simulink model "CellCharacterizationHPPC"  (R2023b)
settings: Solver=ode1be  StartTime=0.0  StopTime=100000  FixedStep=1  MaxStep=1  RelTol=1e-3  AbsTol=1e-3
PreLoadFcn:
  | createHPPCprofile = load('origCellDataHPPCdataGen.mat');
libraries: fl_lib x2, nesl_utility x2, batteryecm_lib x1
settings Model: Creator=The MathWorks, Inc.  LastModifiedBy=jjha
settings SolverCC: AutoScaleAbsTol=off  AlgebraicLoopSolver=TrustRegion  MaxZcPerStep=1
settings DataIOCC: ReturnWorkspaceOutputsName=batt_BatteryCellCharacterizationForBEV_HPPC
settings OptimizationCC: ReuseModelBlockBuffer=off
settings DebuggingCC: UnconnectedInputMsg=warning  UnconnectedOutputMsg=warning  UnconnectedLineMsg=warning  SymbolicDimsDataTypeCodeGenerationDiagnostic=none
settings ModelReferenceCC: EnableRefExpFcnMdlSchedulingChecks=on
settings SFSimCC: CustomCodeUndefinedFunction=UseInterfaceOnly
settings RTWCC: DLArmComputeVersion=19.05
settings SimscapeCC: SimscapeLogType=all  SimscapeLogSimulationStatistics=on  SimscapeLogName=simlog_CellCharacterizationHPPC  SimscapeLogDataHistory=10000

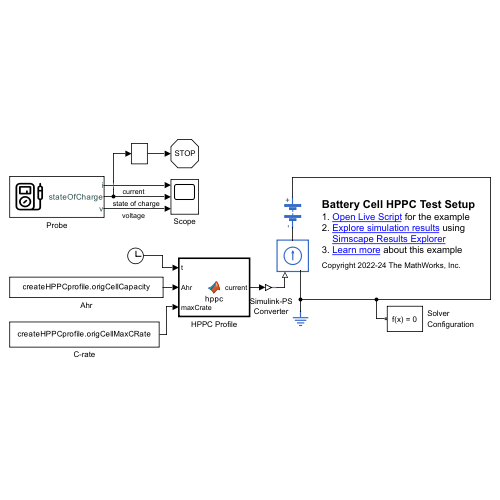
[thumbnail: Simulink's stored preview of the top-level diagram]
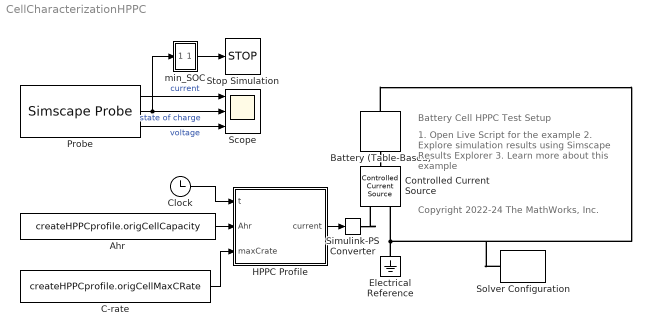
== system CellCharacterizationHPPC ==
  note: Battery Cell HPPC Test Setup
  note: 1. Open Live Script for the example
      | 2. Explore simulation results using
      | Simscape Results Explorer
      | 3. Learn more about this example
  note: Copyright 2022-24 The MathWorks, Inc.
  Ahr : Constant  Value=createHPPCprofile.origCellCapacity
  Battery (Table-Based) : batteryecm_lib/Battery (Table-Based)  SOC_vec=createHPPCprofile.origCellData.SOC  T_dependence=simscape.enum.tablebattery.temperature_dependence.no  prm_dir=simscape.enum.tablebattery.prm_dir.currentDirectionality  T_vec=[278, 293, 313] K  V0_mat=[3.49, 3.5, 3.51; 3.55, 3.57, 3.56; 3.62, 3.63, 3.64; 3.71, 3.71, 3.72; 3.91, 3.93, 3.94; 4.07, 4.08, 4.08; 4.19, 4.19, 4.19] V  V0_vec=createHPPCprofile.origCellData.V0 V  V_range=[0, inf] V  R0_mat=[.0117, .0085, .009; .011, .0085, .009; .0114, .0087, .0092; .0107, .0082, .0088; .0107, .0083, .0091; .0113, .0085, .0089; .0116, .0085, .0089] Ohm  R0_vec=origCell.R0 Ohm  R0_dis_mat=[.0117, .0085, .009; .011, .0085, .009; .0114, .0087, .0092; .0107, .0082, .0088; .0107, .0083, .0091; .0113, .0085, .0089; .0116, .0085, .0089] Ohm  R0_dis_vec=createHPPCprofile.origCellData.R0discharge Ohm  R0_ch_mat=[.0117, .0085, .009; .011, .0085, .009; .0114, .0087, .0092; .0107, .0082, .0088; .0107, .0083, .0091; .0113, .0085, .0089; .0116, .0085, .0089] Ohm  R0_ch_vec=createHPPCprofile.origCellData.R0charge Ohm  AH=createHPPCprofile.origCellCapacity A*hr  prm_leak=simscape.enum.tablebattery.prm_leak.disabled  Rleak_vec=[8000, 7000, 6000] Ohm  Rleak=7e3 Ohm  extrapolation_option=simscape.enum.extrapolation.nearest  SOC_port=simscape.enum.tablebattery.enable.no  prm_dyn=simscape.enum.tablebattery.prm_dyn.rc3  R1_mat=[.0109, .0029, .0013; .0069, .0024, .0012; .0047, .0026, .0013; .0034, .0016, .001; .0033, .0023, .0014; .0033, .0018, .0011; .0028, .0017, .0011] Ohm  R1_vec=createHPPCprofile.origCellData.R1rest Ohm  tau1_mat=[20, 36, 39; 31, 45, 39; 109, 105, 61; 36, 29, 26; 59, 77, 67; 40, 33, 29; 25, 39, 33] s  tau1_vec=createHPPCprofile.origCellData.Tau1rest s  R2_mat=[.0109, .0029, .0013; .0069, .0024, .0012; .0047, .0026, .0013; .0034, .0016, .001; .0033, .0023, .0014; .0033, .0018, .0011; .0028, .0017, .0011] Ohm  R2_vec=createHPPCprofile.origCellData.R2rest Ohm  tau2_mat=[20, 36, 39; 31, 45, 39; 109, 105, 61; 36, 29, 26; 59, 77, 67; 40, 33, 29; 25, 39, 33] s  tau2_vec=createHPPCprofile.origCellData.Tau2rest s  R3_mat=[.0109, .0029, .0013; .0069, .0024, .0012; .0047, .0026, .0013; .0034, .0016, .001; .0033, .0023, .0014; .0033, .0018, .0011; .0028, .0017, .0011] Ohm  R3_vec=createHPPCprofile.origCellData.R3rest Ohm  tau3_mat=[20, 36, 39; 31, 45, 39; 109, 105, 61; 36, 29, 26; 59, 77, 67; 40, 33, 29; 25, 39, 33] s  tau3_vec=createHPPCprofile.origCellData.Tau3rest s  R4_mat=[.0109, .0029, .0013; .0069, .0024, .0012; .0047, .0026, .0013; .0034, .0016, .001; .0033, .0023, .0014; .0033, .0018, .0011; .0028, .0017, .0011] Ohm  R4_vec=[.0029, .0024, .0026, .0016, .0023, .0018, .0017] Ohm  tau4_mat=[20, 36, 39; 31, 45, 39; 109, 105, 61; 36, 29, 26; 59, 77, 67; 40, 33, 29; 25, 39, 33] s  tau4_vec=[36, 45, 105, 29, 77, 33, 39] s  R5_mat=[.0109, .0029, .0013; .0069, .0024, .0012; .0047, .0026, .0013; .0034, .0016, .001; .0033, .0023, .0014; .0033, .0018, .0011; .0028, .0017, .0011] Ohm  R5_vec=[.0029, .0024, .0026, .0016, .0023, .0018, .0017] Ohm  tau5_mat=[20, 36, 39; 31, 45, 39; 109, 105, 61; 36, 29, 26; 59, 77, 67; 40, 33, 29; 25, 39, 33] s  tau5_vec=[36, 45, 105, 29, 77, 33, 39] s  prm_fade=simscape.enum.tablebattery.prm_fade.disabled  N0=100  dV0=0  dR0=0  dAH=0  dRleak=0  dR1=0  dR2=0  dR3=0  dR4=0  dR5=0  N0vec=[100, 200, 300]  Tfadevec=[298.15, 323.15] K  dV0vec=[0, 0, 0]  dR0vec=[0, 0, 0]  dAHvec=[0, 0, 0]  dRleakvec=[0, 0, 0]  dR1vec=[0, 0, 0]  dR2vec=[0, 0, 0]  dR3vec=[0, 0, 0]  dR4vec=[0, 0, 0]  dR5vec=[0, 0, 0]  dV0mat=[0, 0; 0, 0; 0, 0]  dR0mat=[0, 0; 0, 0; 0, 0]  dAHmat=[0, 0; 0, 0; 0, 0]  dRleakmat=[0, 0; 0, 0; 0, 0]  dR1mat=[0, 0; 0, 0; 0, 0]  dR2mat=[0, 0; 0, 0; 0, 0]  dR3mat=[0, 0; 0, 0; 0, 0]  dR4mat=[0, 0; 0, 0; 0, 0]  dR5mat=[0, 0; 0, 0; 0, 0]  prm_age_modeling=simscape.enum.tablebattery.prm_age_modeling.equation  storage_dt_age_vec=[0] d  storage_T_age_vec=[273] K  prm_age_OCV=simscape.enum.tablebattery.prm_age_OCV.OCV  OCV_age=0.9  SOC_age=0.6  prm_age_resistance=simscape.enum.tablebattery.prm_age.disabled  OCV_scaling_age_resistance=2.2134e6  OCV_offset_age_resistance=1.632e6  temp_exp_age_resistance=0.515833569 V  t_exp_age_resistance=0.75  T_age_vec_resistance=[273.15, 298.15, 323.15] K  dt_age_vec_resistance=[90, 180, 270, 360] d  dR0_age_vec=[0, 0, 0]  t_meas_dR0_age=100 d  dR0_age_mat=[0, 0, 0; 0, 0, 0; 0, 0, 0; 0, 0, 0]  prm_age_capacity=simscape.enum.tablebattery.prm_age.disabled  OCV_scaling_age_capacity=1.5097e07  OCV_offset_age_capacity=8.3625e06  temp_exp_age_capacity=0.6011 V  t_exp_age_capacity=0.75  T_age_vec_capacity=[273.15, 298.15, 323.15] K  dt_age_vec_capacity=[90, 180, 270, 360] d  dAH_age_vec=[0, 0, 0]  t_meas_dAH_age=100 d  dAH_age_mat=[0, 0, 0; 0, 0, 0; 0, 0, 0; 0, 0, 0]  thermal_port=simscape.enum.thermaleffects.omit  temperature=298.15 K  thermal_mass=100 J/K  i_specify=off  i_priority=None  i=0 A  i_nominal_specify=off  i_nominal_unit=A  i_nominal_value=1  v_specify=off  v_priority=None  v=0 V  v_nominal_specify=off  v_nominal_unit=V  v_nominal_value=1  stateOfCharge_specify=off  stateOfCharge_priority=High  stateOfCharge=1  stateOfCharge_nominal_specify=off  stateOfCharge_nominal_unit=1  stateOfCharge_nominal_value=1  num_cycles_specify=off  num_cycles_priority=High  num_cycles=0  num_cycles_nominal_specify=off  num_cycles_nominal_unit=1  num_cycles_nominal_value=1  cell_temperature_specify=off  cell_temperature_priority=High  cell_temperature=298.15 K  cell_temperature_nominal_specify=off  cell_temperature_nominal_unit=K  cell_temperature_nominal_value=1
      settings: InternalSimscapePortConfiguration="{\"Bottom\":[],\"Left\":[{\"id\":\"p\",\"label\":\"+\",\"type\":\"foundation.electrical.electrical\"}],\"Right\":[{\"id\":\"n\",\"label\":\"-\",\"type\":\"foundation.electrical.electrical\"}],\"Top\":[]}"
      settings: LibrarySourceBlock=|
      | batt_lib/Cells/Battery
      | (Table-Based)
  C-rate : Constant  Value=createHPPCprofile.origCellMaxCRate
  Clock : Clock
  Controlled Current Source : fl_lib/Electrical/Electrical Sources/Controlled Current Source
  Electrical Reference : fl_lib/Electrical/Electrical Elements/Electrical Reference
  HPPC Profile : MATLAB Function  TreatAsAtomicUnit=on
  Probe : SimscapeProbe  BoundBlock=22  Variables={i, stateOfCharge, v}
  Scope : Scope  NumInputPorts=3
  Simulink-PS Converter : nesl_utility/Simulink-PS Converter  PhysicalDomain=network_engine_domain  SubClassName=ps_input  LeftPortType=input  RightPortType=output  PseudoPeriodic=off  Frequencies=[]  NoiseDistribution=none  NoiseParameters=[]  Unit=A  AffineConversion=off  FilteringAndDerivatives=provide  SimscapeFilterOrder=1  InputFilterTimeConstant=0.001  UdotUserProvided=0
  Solver Configuration : nesl_utility/Solver Configuration  PhysicalDomain=network_engine_domain  SubClassName=solver  LeftPortType=input  RightPortType=generic  Tones=[]  Harmonics=[]  SimulateNoise=off  Profile=off  UseLocalSampling=off  EnableSwitchedLinearOptims=on  FrequencyDomain=off  UseCCode=off  RelTol=0.001  AbsTol=1e-06  MinStep=1e-09  ToWorkspace=off  RevertToSquareIcSolve=off  NumHomotopyIterations=100  PhasorMode=off  PhasorModeNumHarmonics=1  ConsistencySolver=NEWTON_XTOL_AFTER_FTOL  IndexReductionMethod=DerivativeReplacement  DoDC=off  ResidualTolerance=1e-09  ConsistencyTolSource=GLOBAL  ConsistencyAbsTol=0.001  ConsistencyRelTol=0.001  ConsistencyTolFactor=0.001  UseLocalSolver=off  LocalSolverChoice=NE_BACKWARD_EULER_ADVANCER  ResolveIndetEquations=on  FunctionEvalNumThread=1  LocalSolverSampleTime=0.001  DoFixedCost=off  MaxNonlinIter=3  MaxModeIter=2  ComputeImpulses=off  ImpulseIterations=2  LinearAlgebra=auto  LinearAlgebraNumThread=0  EquationFormulation=NE_TIME_EF  DelaysMemoryBudget=1024  AutomaticFiltering=on  FilteringTimeConstant=0.001  PartitionStorageMethod=AS_NEEDED  PartitionMemoryBudget=1024  PartitionMethod=ROBUST  MultibodyUseLocalSolver=off  MultibodyLocalSolverChoice=ODE1  MultibodyLocalSolverSampleTime=0.001
  Stop Simulation : Stop
  min_SOC : Subsystem
  wires:
  Probe/1 -> Scope/1  "current"
  Probe/2 -> min_SOC/1(" "), Scope/2  "state of charge"
  Probe/3 -> Scope/3  "voltage"
  Clock/1 -> HPPC Profile/1(t)
  HPPC Profile/1(current) -> Simulink-PS Converter/1
  Ahr/1 -> HPPC Profile/2(Ahr)
  min_SOC/1("  ") -> Stop Simulation/1
  C-rate/1 -> HPPC Profile/3(maxCrate)
  connections:
  Battery (Table-Based)/RConn1 -- Controlled Current Source/LConn1
  Simulink-PS Converter/RConn1 -- Controlled Current Source/RConn1
  Electrical Reference/LConn1 -- Controlled Current Source/RConn2 -- Solver Configuration/RConn1 -- Battery (Table-Based)/LConn1

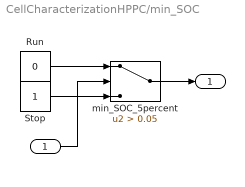
== system CellCharacterizationHPPC/min_SOC ==
  " " : Inport
  Run : Constant  Value=0
  Stop : Constant
  min_SOC_5percent : Switch  Criteria=u2 > Threshold  Threshold=0.05  SaturateOnIntegerOverflow=off  InputSameDT=off
  "  " : Outport
  wires:
  Run/1 -> min_SOC_5percent/1
  Stop/1 -> min_SOC_5percent/3
  " "/1 -> min_SOC_5percent/2
  min_SOC_5percent/1 -> "  "/1

== matlab function CellCharacterizationHPPC/HPPC Profile ==
  data: t input; current output; Ahr input; maxCrate input
function current = hppc(t,Ahr,maxCrate)
    dischg = -1; 
    chg = 1;
    cc_rate = 1/3;
    max_c_rate = maxCrate;
    %% Define HPPC protocol
    Imax = Ahr*max_c_rate; % Cell supplier provided maximum current that 
                           % can be passed through a cell, at a given 
                           % temperature
    const_curr_dischg= Ahr*cc_rate;% C/3 rate for moving to next SOC point
    pulse_chg_mag    = 0.75 * Imax;% Magnitude of charge pulse current
    pulse_dischg_mag = Imax;       % Magnitude of discharge pulse current
    pulse_time_gap   = 40;         % Rest time between charge and discharge 
                                   % pulses, in seconds
    pulse_chg_dur    = 10;         % Duration of charge pulse, in seconds
    pulse_dischg_dur = 30;         % Duration of discharge pulse, in seconds
    rest_time        = 3600;       % 2/3rd hour rest post charge-discharge 
                                   % pulse and constant C/3 discharge to the 
                                   % next SOC point 
    soc_sweep_dur    = 900;        % Duration of SOC sweep at cc_rate, in 
                                   % seconds

    %% Generate current
    % Sequence:
    %         t1 = pulse_dischg_dur (discharge pulse)
    %         t2 = pulse_time_gap   (time before next pulse)
    %         t3 = pulse_chg_dur    (charge pulse)
    %         t4 = pulse_time_gap   (time before SOC sweep)
    %         t5 ~ 10% SOC reduction
    %            = 1/3rd of an hour at C/3 rate
    %            = 9% SOC sweep in soc_sweep_dur time
    %         t6 = rest time 
    % Start pulses from ~95% SOC and go upto ~10% SOC

    t_start = 3600 * (0.05 * Ahr) / (cc_rate * Ahr);
    t1 = pulse_dischg_dur; 
    t2 = t1 + pulse_time_gap;
    t3 = t2 + pulse_chg_dur;
    t4 = t3 + pulse_time_gap;
    t5 = t4 + soc_sweep_dur;
    t6 = t5 + rest_time;
    t_oneChgDisch    = pulse_dischg_dur + ...
                       pulse_time_gap + ...
                       pulse_chg_dur + ...
                       pulse_time_gap + ...
                       soc_sweep_dur + ...
                       rest_time;
    if t > t_start + rest_time
        t0 = t - (t_start + rest_time);
        ts = mod(t0,t_oneChgDisch);
        if ts <= t1
            % Discharge pulse
            current = dischg * pulse_dischg_mag;
        elseif ts > t1 && ts <= t2
            % relax after discharge
            current = 0;
        elseif ts > t2 && ts <= t3
            % Charge pulse
            current = chg * pulse_chg_mag;
        elseif ts > t3 && ts<= t4
            % Relax after charge
            current = 0;
        elseif ts > t4 && ts <= t5
            % SOC sweep
            current = dischg * Ahr * cc_rate;
        else
            % Rest
            current = 0;
        end
    else
        if t < t_start
            current = dischg * cc_rate * Ahr;
        else
            current = 0;
        end
    end

    current = (-1) * current;
end
